simulink model "ArcIndex"  (R2018b)
settings: Solver=VariableStepAuto  StartTime=0.0  StopTime=86400  RelTol=1e-3  EnableMultiTasking=on
undefined symbols (not defined in the file): DiffuseHorizontal, DNI, Wall_Irradiance_Angles_NEWS
libraries: dspindex x3
settings Model: Creator=cpp14rcj  LastModifiedBy=cpp14rcj
settings DataIOCC: LimitDataPoints=on
settings OptimizationCC: LifeSpan=inf
settings DebuggingCC: AllowSymbolicDim=off  SFUnexpectedBacktrackingDiag=warning  SFNoUnconditionalDefaultTransitionDiag=warning  SFExecutionAtInitializationDiag=none
settings ModelReferenceCC: PropagateSignalLabelsOutOfModel=off
settings SFSimCC: SimUseLocalCustomCode=off
settings RTWCC: RTWUseLocalCustomCode=off
settings CodeAppCC: StateflowObjectComments=on
settings GRTTargetCC: TargetLangStandard=C89/C90 (ANSI)
settings ConfigComp: CovMetricSettings=dw  CovHtmlReporting=on  CovSaveCumulativeToWorkspaceVar=on  CovSaveSingleToWorkspaceVar=on  CovExternalEMLEnable=off
settings SimscapeCC: SimscapeNormalizeSystem=off
settings ConfigurationSet: Description=SimMechanics 2G

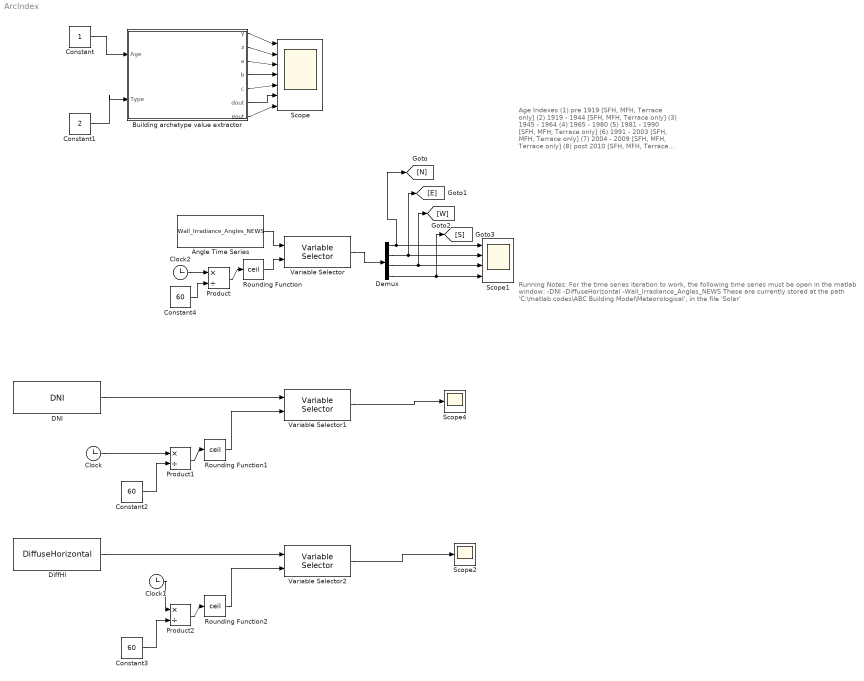
== system ArcIndex ==
  note: Running Notes:
      |
      | For the time series iteration to work, the following time series must be open in the matlab window:
      |
      | -DNI
      |
      | -DiffuseHorizontal
      |
      | -Wall_Irradiance_Angles_NEWS
      |
      | These are currently stored at the path 'C:\matlab codes\ABC Building Model\Meteorological', in the file 'Solar'
  note: Age Indexes
      |
      | (1) pre 1919 [SFH, MFH, Terrace only]
      | (2) 1919 - 1944 [SFH, MFH, Terrace only]
      | (3) 1945 - 1964
      | (4) 1965 - 1980
      | (5) 1981 - 1990 [SFH, MFH, Terrace only]
      | (6) 1991 - 2003 [SFH, MFH, Terrace only]
      | (7) 2004 - 2009 [SFH, MFH, Terrace only]
      | (8) post 2010 [SFH, MFH, Terrace only]
      | (9) post 2004 [Apartment only]
      |
      | Type Indexes
      |
      | (1) SFH '
      | (2) Terraced house'
      | (3) MFH '
      | (4) Apartment
  Angle Time Series : Constant  Value=Wall_Irradiance_Angles_NEWS
  Building archetype value extractor : MATLAB Function  TreatAsAtomicUnit=on
  Clock : Clock
  Clock1 : Clock
  Clock2 : Clock
  Constant : Constant
  Constant1 : Constant  Value=2
  Constant2 : Constant  Value=60
  Constant3 : Constant  Value=60
  Constant4 : Constant  Value=60
  DNI : Constant  Value=DNI
  Demux : Demux
  DiffHI : Constant  Value=DiffuseHorizontal
  Product : Product  Inputs=*/
  Product1 : Product  Inputs=*/
  Product2 : Product  Inputs=*/
  Rounding Function : Rounding  Operator=ceil
  Rounding Function1 : Rounding  Operator=ceil
  Rounding Function2 : Rounding  Operator=ceil
  Scope : Scope  NumInputPorts=7
  Scope1 : Scope  NumInputPorts=4
  Scope2 : Scope
  Scope4 : Scope
  Variable Selector : dspindex/Variable Selector  NumInputs=1  rowsOrCols=Rows  IdxMode=Variable  Elements=[1 3]  ZerOneIdxMode=One-based  errmode=Clip Index  FillMode=on  FillValues=0
  Variable Selector1 : dspindex/Variable Selector  NumInputs=1  rowsOrCols=Rows  IdxMode=Variable  Elements=[1 3]  ZerOneIdxMode=One-based  errmode=Clip Index  FillMode=on  FillValues=0
  Variable Selector2 : dspindex/Variable Selector  NumInputs=1  rowsOrCols=Rows  IdxMode=Variable  Elements=[1 3]  ZerOneIdxMode=One-based  errmode=Clip Index  FillMode=on  FillValues=0
  wires:
  Constant/1 -> Building archetype value extractor/1(Age)
  Constant1/1 -> Building archetype value extractor/2(Type)
  Building archetype value extractor/1(y) -> Scope/1
  Building archetype value extractor/2(z) -> Scope/2
  Building archetype value extractor/3(a) -> Scope/3
  Building archetype value extractor/4(b) -> Scope/4
  Building archetype value extractor/5(c) -> Scope/5
  Building archetype value extractor/6(dout) -> Scope/6
  Building archetype value extractor/7(eout) -> Scope/7
  Rounding Function/1 -> Variable Selector/2
  Angle Time Series/1 -> Variable Selector/1
  Variable Selector/1 -> Demux/1
  Demux/1 -> Scope1/1, [N]
  Demux/4 -> Scope1/4, [S]
  Clock2/1 -> Product/1
  Product/1 -> Rounding Function/1
  Constant4/1 -> Product/2
  Demux/2 -> [E], Scope1/2
  Demux/3 -> [W], Scope1/3
  Rounding Function1/1 -> Variable Selector1/2
  DNI/1 -> Variable Selector1/1
  Variable Selector1/1 -> Scope4/1
  Clock/1 -> Product1/1
  Product1/1 -> Rounding Function1/1
  Constant2/1 -> Product1/2
  Rounding Function2/1 -> Variable Selector2/2
  DiffHI/1 -> Variable Selector2/1
  Variable Selector2/1 -> Scope2/1
  Clock1/1 -> Product2/1
  Product2/1 -> Rounding Function2/1
  Constant3/1 -> Product2/2

== matlab function ArcIndex/Building archetype value extractor ==
  data: Age input; y output double size=[1 1]; Type input; z output; a output; b output; c output; dout output; eout output
function [y, z, a, b, c, dout, eout] = ArcIndex(Age, Type)

AgeVector={'pre 1919';'1919 - 1944';'1945 - 1964';'1965  - 1980';'1981 - 1990';'1991 - 2003';'2004 - 2009';'post 2010';'pre 1919';'1919 - 1944';'1945 - 1964';'1965  - 1980';'1981 - 1990';'1991 - 2003';'2004 - 2009';'post 2010';'pre 1919';'1919 - 1944';'1945 - 1964';'1965  - 1980';'1981 - 1990';'1991 - 2003';'2004 - 2009';'post 2010';'pre 1919';'1919 - 1944';'1945 - 1964';'1965  - 1980';'1981 - 1990';'1991 - 2003';'post 2004'}

TypeVector={'SFH';'SFH';'SFH';'SFH';'SFH';'SFH';'SFH';'SFH';'Terraced house';'Terraced house';'Terraced house';'Terraced house';'Terraced house';'Terraced house';'Terraced house';'Terraced house';'MFH';'MFH';'MFH';'MFH';'MFH';'MFH';'MFH';'MFH';'Apartment';'Apartment';'Apartment';'Apartment';'Apartment';'Apartment';'Apartment'};

UVals_Archetypes=[2.30000000000000,2.10000000000000,0.720000000000000,4.80000000000000,3,0.562500000000000,3.80000000000000;2.30000000000000,2.10000000000000,0.720000000000000,4.80000000000000,3,0.775000000000000,3.80000000000000;2.30000000000000,1.60000000000000,0.720000000000000,4.80000000000000,3,0.760000000000000,3.80000000000000;1.50000000000000,1.60000000000000,0.720000000000000,3.10000000000000,2,0.725000000000000,3.80000000000000;0.400000000000000,1.60000000000000,0.720000000000000,3.10000000000000,2,0.495000000000000,3.80000000000000;0.400000000000000,1.60000000000000,0.500000000000000,3.10000000000000,2,0.510000000000000,3.80000000000000;0.250000000000000,0.350000000000000,0.250000000000000,1.85000000000000,2,0.350000000000000,3.80000000000000;0.180000000000000,0.280000000000000,0.220000000000000,1.85000000000000,2,0.350000000000000,3.80000000000000;2.30000000000000,2.10000000000000,0.590000000000000,4.80000000000000,3,0.562500000000000,3.80000000000000;2.30000000000000,2.10000000000000,0.590000000000000,4.80000000000000,3,0.775000000000000,3.80000000000000;2.30000000000000,1.60000000000000,0.590000000000000,4.80000000000000,3,0.760000000000000,3.80000000000000;1.50000000000000,1.60000000000000,0.590000000000000,3.10000000000000,2,0.725000000000000,3.80000000000000;0.400000000000000,1.60000000000000,0.590000000000000,3.10000000000000,2,0.495000000000000,3.80000000000000;0.400000000000000,1.60000000000000,0.500000000000000,3.10000000000000,2,0.510000000000000,3.80000000000000;0.250000000000000,0.350000000000000,0.250000000000000,1.85000000000000,2,0.350000000000000,3.80000000000000;0.180000000000000,0.280000000000000,0.220000000000000,1.85000000000000,2,0.350000000000000,3.80000000000000;2.30000000000000,2.10000000000000,0.450000000000000,4.80000000000000,3,0.562500000000000,3.80000000000000;2.30000000000000,2.10000000000000,0.450000000000000,4.80000000000000,3,0.775000000000000,3.80000000000000;2.30000000000000,1.60000000000000,0.450000000000000,4.80000000000000,3,0.760000000000000,3.80000000000000;1.50000000000000,1.60000000000000,0.450000000000000,3.10000000000000,2,0.725000000000000,3.80000000000000;0.400000000000000,1.60000000000000,0.450000000000000,3.10000000000000,2,0.495000000000000,3.80000000000000;0.400000000000000,1.60000000000000,0.500000000000000,3.10000000000000,2,0.510000000000000,3.80000000000000;0.250000000000000,0.350000000000000,0.250000000000000,1.85000000000000,2,0.350000000000000,3.80000000000000;0.180000000000000,0.280000000000000,0.220000000000000,1.85000000000000,2,0.350000000000000,3.80000000000000;NaN,NaN,NaN,NaN,NaN,NaN,NaN;NaN,NaN,NaN,NaN,NaN,NaN,NaN;2.30000000000000,2.10000000000000,0.450000000000000,4.80000000000000,3,0.760000000000000,3.80000000000000;1.30000000000000,1.60000000000000,0.450000000000000,3.10000000000000,2,0.725000000000000,3.80000000000000;NaN,NaN,NaN,NaN,NaN,NaN,NaN;NaN,NaN,NaN,NaN,NaN,NaN,NaN;0.250000000000000,0.350000000000000,0.220000000000000,1.85000000000000,2,0.350000000000000,3.80000000000000];


Alookup=['pre 1919   '
 '1919 - 1944'
 '1945 - 1964'
 '1965 - 1980'
 '1981 - 1990'
 '1991 - 2003'
 '2004 - 2009'
 'post 2010  '
 'post 2004  ']
Tlookup=['SFH           '
 'Terraced house'
 'MFH           '
 'Apartment     '];


d=['pre 1919    '
'1919 - 1944 '
'1945 - 1964 '
'1965  - 1980'
'1981 - 1990 '
'1991 - 2003 '
'2004 - 2009 '
'post 2010   '
'pre 1919    '
'1919 - 1944 '
'1945 - 1964 '
'1965  - 1980'
'1981 - 1990 '
'1991 - 2003 '
'2004 - 2009 '
'post 2010   '
'pre 1919    '
'1919 - 1944 '
'1945 - 1964 '
'1965  - 1980'
'1981 - 1990 '
'1991 - 2003 '
'2004 - 2009 '
'post 2010   '
'pre 1919    '
'1919 - 1944 '
'1945 - 1964 '
'1965  - 1980'
'1981 - 1990 '
'1991 - 2003 '
'post 2004   ']


e=['SFH           '
'SFH           '
'SFH           '
'SFH           '
'SFH           '
'SFH           '
'SFH           '
'SFH           '
'Terraced house'
'Terraced house'
'Terraced house'
'Terraced house'
'Terraced house'
'Terraced house'
'Terraced house'
'Terraced house'
'MFH           '
'MFH           '
'MFH           '
'MFH           '
'MFH           '
'MFH           '
'MFH           '
'MFH           '
'Apartment     '
'Apartment     '
'Apartment     '
'Apartment     '
'Apartment     '
'Apartment     '
'Apartment     ']



[~,index] = ismember(d,Alookup(Age,:),'rows');
k=find(index);

[~,index2] = ismember(e,Tlookup(Type,:),'rows');
m=find(index2);

p=intersect(k,m);
p(p==0)=[];
p=p(1,1);

y=UVals_Archetypes(p,1);
z=UVals_Archetypes(p,2);
a=UVals_Archetypes(p,3);
b=UVals_Archetypes(p,4);
c=UVals_Archetypes(p,5);
dout=UVals_Archetypes(p,6);
eout=UVals_Archetypes(p,7);

end

%%
